simulink model "L1_CBF_ACC"  (R2018a)
settings: Solver=FixedStepAuto  StartTime=0.0  StopTime=Tsim  FixedStep=0.001  RelTol=1e-3
InitFcn:
  | tic;
  | disp('Simulation started...');
  | L1_CBF_ACC
StopFcn:
  | elapsedTime_L1 = toc; % Stop timer when simulation ends
  | fprintf('Simulation Time: %.6f seconds\n', elapsedTime_L1);
  | 
  | % out_L1 = out;
undefined symbols (not defined in the file): case_num, D0, epsilon, f0, f1, f2, g, gamma, GTP, k, k_fric, m, magnitude, omega0, p_omega, psc, v0, vd, x10, x20
libraries: Projection x2
settings Model: Creator=Administrator  LastModifiedBy=hieunguyen412
settings DataIOCC: ReturnWorkspaceOutputs=on
settings SFSimCC: SimUseLocalCustomCode=on
settings RTWCC: RTWUseLocalCustomCode=on

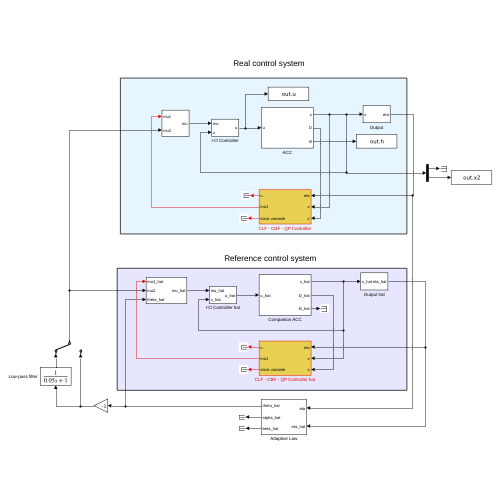
[thumbnail: Simulink's stored preview of the top-level diagram]
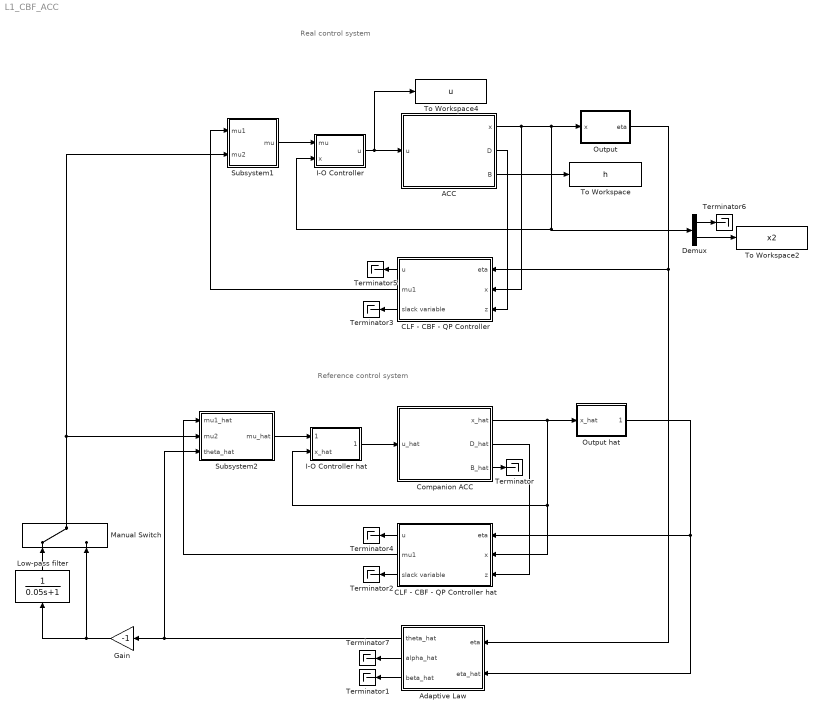
== system L1_CBF_ACC ==
  note: Real control system
  note: Reference control system
  ACC : Subsystem
  Adaptive Law : Subsystem
  CLF - CBF - QP Controller : Subsystem
  CLF - CBF - QP Controller hat : Subsystem
  Companion ACC : Subsystem
  Demux : Demux  Outputs=2
  Gain : Gain  Gain=-1
  I-O Controller : Subsystem
  I-O Controller hat : Subsystem
  Low-pass filter : TransferFcn  Denominator=[0.05 1]
  Manual Switch : ManualSwitch
  Output : Subsystem
  Output hat : Subsystem
  Subsystem1 : Subsystem
  Subsystem2 : Subsystem
  Terminator{,1..7} (8 alike) : Terminator
  To Workspace : ToWorkspace  VariableName=h  SampleTime=-1
  To Workspace2 : ToWorkspace  VariableName=x2  SampleTime=-1
  To Workspace4 : ToWorkspace  VariableName=u  SampleTime=-1
  wires:
  ACC/1(x) -> CLF - CBF - QP Controller/2(x), I-O Controller/2(x), Demux/1, Output/1(x)
  Output/1(eta) -> Adaptive Law/1(eta), CLF - CBF - QP Controller/1(eta)
  I-O Controller/1(u) -> To Workspace4/1, ACC/1(u)
  Adaptive Law/2(alpha_hat) -> Terminator7/1
  Adaptive Law/3(beta_hat) -> Terminator1/1
  ACC/3(B) -> To Workspace/1
  CLF - CBF - QP Controller/3(slack variable) -> Terminator3/1
  CLF - CBF - QP Controller/1(u) -> Terminator5/1
  ACC/2(D) -> CLF - CBF - QP Controller/3(z)
  Demux/2 -> To Workspace2/1
  Demux/1 -> Terminator6/1
  Subsystem1/1(mu) -> I-O Controller/1(mu)
  CLF - CBF - QP Controller/2(mu1) -> Subsystem1/1(mu1)
  CLF - CBF - QP Controller hat/2(mu1) -> Subsystem2/1(mu1_hat)
  Subsystem2/1(mu_hat) -> I-O Controller hat/1(mu_hat)
  Companion ACC/2(D_hat) -> CLF - CBF - QP Controller hat/3(z)
  CLF - CBF - QP Controller hat/1(u) -> Terminator4/1
  CLF - CBF - QP Controller hat/3(slack variable) -> Terminator2/1
  I-O Controller hat/1(u_hat) -> Companion ACC/1(u_hat)
  Output hat/1(eta_hat) -> Adaptive Law/2(eta_hat), CLF - CBF - QP Controller hat/1(eta)
  Companion ACC/1(x_hat) -> CLF - CBF - QP Controller hat/2(x), I-O Controller hat/2(x_hat), Output hat/1(x_hat)
  Low-pass filter/1 -> Manual Switch/1
  Gain/1 -> Low-pass filter/1, Manual Switch/2
  Manual Switch/1 -> Subsystem1/2(mu2), Subsystem2/2(mu2)
  Adaptive Law/1(theta_hat) -> Gain/1, Subsystem2/3(theta_hat)
  Companion ACC/3(B_hat) -> Terminator/1

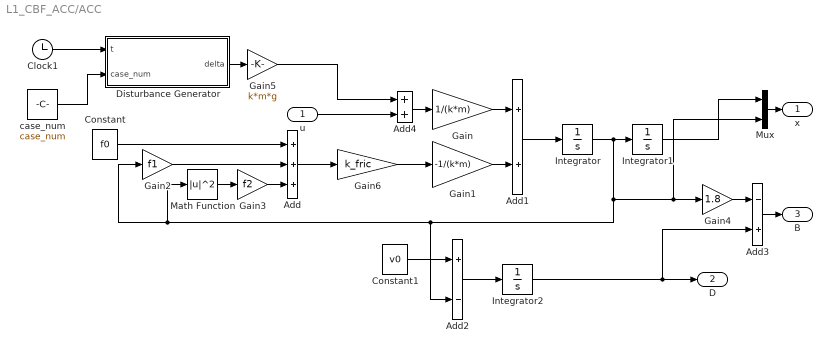
== system L1_CBF_ACC/ACC ==
  u : Inport  PortDimensions=1
  Add : Sum  Inputs=+++
  Add1 : Sum
  Add2 : Sum  Inputs=+-
  Add3 : Sum  Inputs=-+
  Add4 : Sum
  Clock1 : Clock
  Constant : Constant  Value=f0
  Constant1 : Constant  Value=v0
  Disturbance Generator : MATLAB Function  TreatAsAtomicUnit=on
  Gain : Gain  Gain=1/(k*m)
  Gain1 : Gain  Gain=-1/(k*m)
  Gain2 : Gain  Gain=f1
  Gain3 : Gain  Gain=f2
  Gain4 : Gain  Gain=1.8
  Gain5 : Gain  Gain=k*m*g
  Gain6 : Gain  Gain=k_fric
  Integrator : Integrator  InitialCondition=x20
  Integrator1 : Integrator  InitialCondition=x10
  Integrator2 : Integrator  InitialCondition=D0
  Math Function : Math  Operator=magnitude^2  SaturateOnIntegerOverflow=on
  Mux : Mux  Inputs=2
  case_num : Constant  Value=case_num
  x : Outport  PortDimensions=2
  D : Outport  Port=2  PortDimensions=1
  B : Outport  Port=3  PortDimensions=1
  wires:
  Constant/1 -> Add/1
  Gain2/1 -> Add/2
  Gain3/1 -> Add/3
  Gain/1 -> Add1/1
  Gain1/1 -> Add1/2
  Add1/1 -> Integrator/1
  Integrator/1 -> Add2/2, Math Function/1, Gain2/1, Mux/2, Gain4/1, Integrator1/1
  Math Function/1 -> Gain3/1
  Constant1/1 -> Add2/1
  Add2/1 -> Integrator2/1
  Integrator2/1 -> Add3/2, D/1
  Gain4/1 -> Add3/1
  Add3/1 -> B/1
  Mux/1 -> x/1
  Integrator1/1 -> Mux/1
  Gain5/1 -> Add4/1
  Add4/1 -> Gain/1
  Add/1 -> Gain6/1
  Gain6/1 -> Gain1/1
  u/1 -> Add4/2
  case_num/1 -> Disturbance Generator/2(case_num)
  Clock1/1 -> Disturbance Generator/1(t)
  Disturbance Generator/1(delta) -> Gain5/1

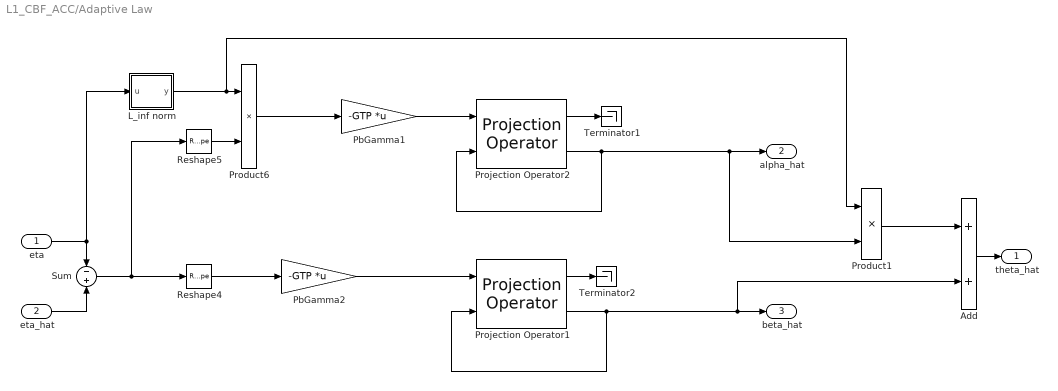
== system L1_CBF_ACC/Adaptive Law ==
  eta : Inport
  eta_hat : Inport  Port=2
  Add : Sum
  L_inf norm : MATLAB Function  TreatAsAtomicUnit=on
  PbGamma1 : Gain  Gain=-GTP  Multiplication=Matrix(K*u) (u vector)
  PbGamma2 : Gain  Gain=-GTP  Multiplication=Matrix(K*u) (u vector)
  Product1 : Product  RndMeth=Zero
  Product6 : Product  RndMeth=Zero
  Projection Operator1 : Projection/Projection Operator  EpsilonTheta=epsilon_beta  Prmax=beta_max  Prcenter=0  Pr0=0
  Projection Operator2 : Projection/Projection Operator  EpsilonTheta=epsilon_alpha  Prmax=alpha_max  Prcenter=0  Pr0=0
  Reshape4 : Reshape  OutputDimensionality=Row vector (2-D)
  Reshape5 : Reshape  OutputDimensionality=Row vector (2-D)
  Sum : Sum  Inputs=-+
  Terminator1 : Terminator
  Terminator2 : Terminator
  theta_hat : Outport
  alpha_hat : Outport  Port=2
  beta_hat : Outport  Port=3
  wires:
  Reshape4/1 -> PbGamma2/1
  Reshape5/1 -> Product6/2
  Projection Operator2/1 -> Terminator1/1
  Sum/1 -> Reshape5/1, Reshape4/1
  eta_hat/1 -> Sum/2
  Projection Operator1/1 -> Terminator2/1
  Projection Operator2/2 -> Product1/2, alpha_hat/1, Projection Operator2/2
  Projection Operator1/2 -> Projection Operator1/2, Add/2, beta_hat/1
  PbGamma2/1 -> Projection Operator1/1
  PbGamma1/1 -> Projection Operator2/1
  Product6/1 -> PbGamma1/1
  eta/1 -> Sum/1, L_inf norm/1(u)
  L_inf norm/1(y) -> Product1/1, Product6/1
  Product1/1 -> Add/1
  Add/1 -> theta_hat/1

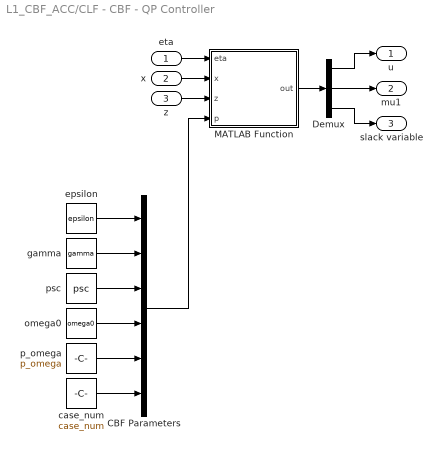
== system L1_CBF_ACC/CLF - CBF - QP Controller ==
  eta : Inport  PortDimensions=1
  x : Inport  Port=2  PortDimensions=2
  z : Inport  Port=3  PortDimensions=1
  CBF Parameters : Mux  Inputs=6
  Demux : Demux  Outputs=3
  MATLAB Function : MATLAB Function  TreatAsAtomicUnit=on  SystemSampleTime=0.001
  case_num : Constant  Value=case_num
  epsilon : Constant  Value=epsilon
  gamma : Constant  Value=gamma
  omega0 : Constant  Value=omega0
  p_omega : Constant  Value=p_omega
  psc : Constant  Value=psc
  u : Outport  PortDimensions=1
  mu1 : Outport  Port=2  PortDimensions=1
  slack variable : Outport  Port=3  PortDimensions=1
  wires:
  Demux/1 -> u/1
  MATLAB Function/1(out) -> Demux/1
  Demux/3 -> slack variable/1
  Demux/2 -> mu1/1
  eta/1 -> MATLAB Function/1(eta)
  x/1 -> MATLAB Function/2(x)
  z/1 -> MATLAB Function/3(z)
  gamma/1 -> CBF Parameters/2
  omega0/1 -> CBF Parameters/4
  epsilon/1 -> CBF Parameters/1
  p_omega/1 -> CBF Parameters/5
  psc/1 -> CBF Parameters/3
  CBF Parameters/1 -> MATLAB Function/4(p)
  case_num/1 -> CBF Parameters/6

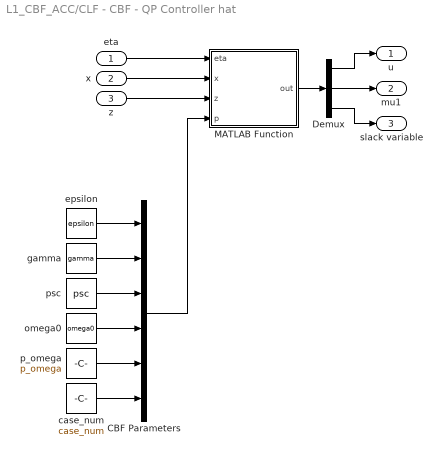
== system L1_CBF_ACC/CLF - CBF - QP Controller hat ==
  eta : Inport  PortDimensions=1
  x : Inport  Port=2  PortDimensions=2
  z : Inport  Port=3  PortDimensions=1
  CBF Parameters : Mux  Inputs=6
  Demux : Demux  Outputs=3
  MATLAB Function : MATLAB Function  TreatAsAtomicUnit=on  SystemSampleTime=0.001
  case_num : Constant  Value=case_num
  epsilon : Constant  Value=epsilon
  gamma : Constant  Value=gamma
  omega0 : Constant  Value=omega0
  p_omega : Constant  Value=p_omega
  psc : Constant  Value=psc
  u : Outport  PortDimensions=1
  mu1 : Outport  Port=2  PortDimensions=1
  slack variable : Outport  Port=3  PortDimensions=1
  wires:
  x/1 -> MATLAB Function/2(x)
  z/1 -> MATLAB Function/3(z)
  eta/1 -> MATLAB Function/1(eta)
  Demux/3 -> slack variable/1
  Demux/2 -> mu1/1
  MATLAB Function/1(out) -> Demux/1
  Demux/1 -> u/1
  case_num/1 -> CBF Parameters/6
  CBF Parameters/1 -> MATLAB Function/4(p)
  p_omega/1 -> CBF Parameters/5
  epsilon/1 -> CBF Parameters/1
  omega0/1 -> CBF Parameters/4
  psc/1 -> CBF Parameters/3
  gamma/1 -> CBF Parameters/2

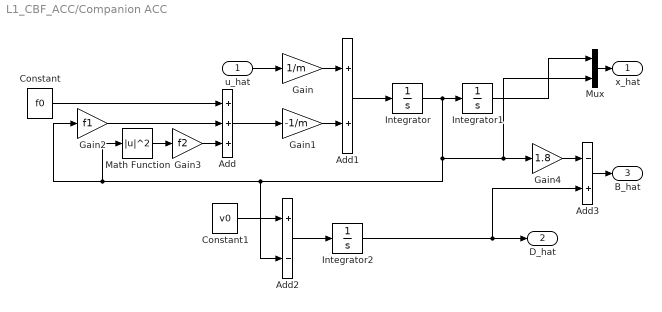
== system L1_CBF_ACC/Companion ACC ==
  u_hat : Inport  PortDimensions=1
  Add : Sum  Inputs=+++
  Add1 : Sum
  Add2 : Sum  Inputs=+-
  Add3 : Sum  Inputs=-+
  Constant : Constant  Value=f0
  Constant1 : Constant  Value=v0
  Gain : Gain  Gain=1/m
  Gain1 : Gain  Gain=-1/m
  Gain2 : Gain  Gain=f1
  Gain3 : Gain  Gain=f2
  Gain4 : Gain  Gain=1.8
  Integrator : Integrator  InitialCondition=x20
  Integrator1 : Integrator  InitialCondition=x10
  Integrator2 : Integrator  InitialCondition=D0
  Math Function : Math  Operator=magnitude^2  SaturateOnIntegerOverflow=on
  Mux : Mux  Inputs=2
  x_hat : Outport  PortDimensions=2
  D_hat : Outport  Port=2  PortDimensions=1
  B_hat : Outport  Port=3  PortDimensions=1
  wires:
  Integrator1/1 -> Mux/1
  Mux/1 -> x_hat/1
  Add3/1 -> B_hat/1
  Gain4/1 -> Add3/1
  Integrator2/1 -> D_hat/1, Add3/2
  Add2/1 -> Integrator2/1
  Constant1/1 -> Add2/1
  Math Function/1 -> Gain3/1
  Integrator/1 -> Mux/2, Gain4/1, Gain2/1, Math Function/1, Add2/2, Integrator1/1
  Add1/1 -> Integrator/1
  Gain1/1 -> Add1/2
  Gain/1 -> Add1/1
  u_hat/1 -> Gain/1
  Gain3/1 -> Add/3
  Gain2/1 -> Add/2
  Constant/1 -> Add/1
  Add/1 -> Gain1/1

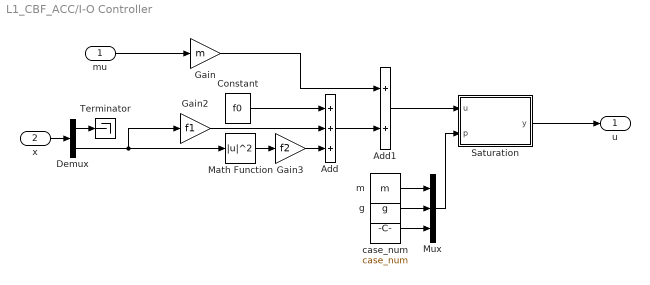
== system L1_CBF_ACC/I-O Controller ==
  mu : Inport
  x : Inport  Port=2  PortDimensions=2
  Add : Sum  Inputs=+++
  Add1 : Sum
  Constant : Constant  Value=f0
  Demux : Demux  Outputs=2
  Gain : Gain  Gain=m
  Gain2 : Gain  Gain=f1
  Gain3 : Gain  Gain=f2
  Math Function : Math  Operator=magnitude^2  SaturateOnIntegerOverflow=on
  Mux : Mux  Inputs=3
  Saturation : MATLAB Function  TreatAsAtomicUnit=on
  Terminator : Terminator
  case_num : Constant  Value=case_num
  g : Constant  Value=g
  m : Constant  Value=m
  u : Outport  PortDimensions=1
  wires:
  Gain3/1 -> Add/3
  Constant/1 -> Add/1
  Math Function/1 -> Gain3/1
  Gain2/1 -> Add/2
  Add/1 -> Add1/2
  mu/1 -> Gain/1
  Gain/1 -> Add1/1
  x/1 -> Demux/1
  Demux/2 -> Math Function/1, Gain2/1
  Demux/1 -> Terminator/1
  Add1/1 -> Saturation/1(u)
  Saturation/1(y) -> u/1
  case_num/1 -> Mux/3
  Mux/1 -> Saturation/2(p)
  g/1 -> Mux/2
  m/1 -> Mux/1

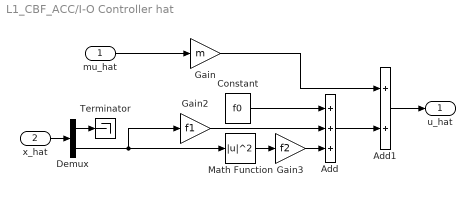
== system L1_CBF_ACC/I-O Controller hat ==
  mu_hat : Inport
  x_hat : Inport  Port=2  PortDimensions=2
  Add : Sum  Inputs=+++
  Add1 : Sum
  Constant : Constant  Value=f0
  Demux : Demux  Outputs=2
  Gain : Gain  Gain=m
  Gain2 : Gain  Gain=f1
  Gain3 : Gain  Gain=f2
  Math Function : Math  Operator=magnitude^2  SaturateOnIntegerOverflow=on
  Terminator : Terminator
  u_hat : Outport  PortDimensions=1
  wires:
  Demux/1 -> Terminator/1
  Demux/2 -> Gain2/1, Math Function/1
  x_hat/1 -> Demux/1
  Add1/1 -> u_hat/1
  Gain/1 -> Add1/1
  mu_hat/1 -> Gain/1
  Add/1 -> Add1/2
  Gain2/1 -> Add/2
  Math Function/1 -> Gain3/1
  Constant/1 -> Add/1
  Gain3/1 -> Add/3

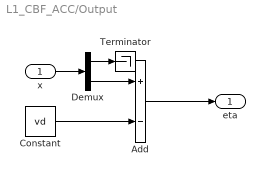
== system L1_CBF_ACC/Output ==
  x : Inport  PortDimensions=2
  Add : Sum  Inputs=+-
  Constant : Constant  Value=vd
  Demux : Demux  Outputs=2
  Terminator : Terminator
  eta : Outport  PortDimensions=1
  wires:
  Constant/1 -> Add/2
  Add/1 -> eta/1
  Demux/2 -> Add/1
  x/1 -> Demux/1
  Demux/1 -> Terminator/1

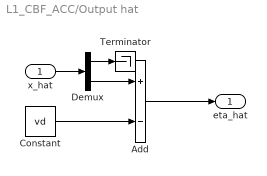
== system L1_CBF_ACC/Output hat ==
  x_hat : Inport  PortDimensions=2
  Add : Sum  Inputs=+-
  Constant : Constant  Value=vd
  Demux : Demux  Outputs=2
  Terminator : Terminator
  eta_hat : Outport  PortDimensions=1
  wires:
  Demux/1 -> Terminator/1
  x_hat/1 -> Demux/1
  Demux/2 -> Add/1
  Add/1 -> eta_hat/1
  Constant/1 -> Add/2

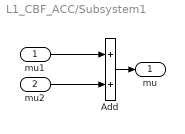
== system L1_CBF_ACC/Subsystem1 ==
  mu1 : Inport
  mu2 : Inport  Port=2
  Add : Sum
  mu : Outport
  wires:
  mu1/1 -> Add/1
  mu2/1 -> Add/2
  Add/1 -> mu/1

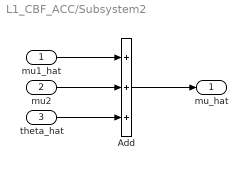
== system L1_CBF_ACC/Subsystem2 ==
  mu1_hat : Inport
  mu2 : Inport  Port=2
  theta_hat : Inport  Port=3
  Add : Sum  Inputs=+++
  mu_hat : Outport
  wires:
  theta_hat/1 -> Add/3
  mu2/1 -> Add/2
  mu1_hat/1 -> Add/1
  Add/1 -> mu_hat/1

== matlab function L1_CBF_ACC/Adaptive Law/L_inf norm ==
  data: u input; y output
function y = fcn(u)

y = max(abs(u));

== matlab function L1_CBF_ACC/I-O Controller/Saturation ==
  data: u input; y output; p input
function y = fcn(u, p)

m = p(1);
g = p(2);
case_num = p(3);

if case_num == 1 || case_num == 2
    y = u;
else
    if u >= 0.3*m*g
        y = 0.3*m*g;
    elseif u <= -0.3*m*g
        y = -0.3*m*g;
    else
        y = u;
    end
end

end

== matlab function L1_CBF_ACC/CLF - CBF - QP Controller hat/MATLAB Function ==
  data: eta input; out output; x input; z input; p input
function out = QP_Controller(eta, x, z, p)
coder.extrinsic('quadprog');

out = zeros(3,1);

x2 = x(2); 

case_num = p(6);
if case_num == 1 || case_num == 2
    mode = 1;
else 
    mode = 2;
end

%% Physical parameters
m = 1650;
g = 9.81; 
f0 = 0.1;
f1 = 5;
f2 = 0.25;
vd = 24;
v0 =  13.89;

ca = 0.3;
cd = 0.3;

%% Controller parameters
epsilon = p(1); 
gamma = p(2);
psc = p(3);
omega0 = p(4); 
p_omega = p(5);

%% Aerodynamic drag force
Fr = f0 + f1*x2 + f2*x2.^2;

%% ============== QP 1 (No input saturation) ==============
if mode == 1
    %% CLF
    y = eta;
    V = y^2;
    LfV = 2*y*(-Fr/m); LgV = 2*y/m;
    A_clf = [LgV 0 -1]; b_clf = -LfV -epsilon*V;
    
    %% CBF
    B = z - 1.8*x2;
    LfB = v0 - x2 + 1.8*Fr/m;
    LgB = -1.8/m;
    A_cbf = [-LgB, 0, 0]; b_cbf = LfB + gamma*B;
    
    %% I-O L
    Lfy = -Fr/m; Lgy = 1/m;
    A_iol = [Lgy -1 0]; b_iol = - Lfy;
    
    %% QP
    A_ieq = [A_clf; A_cbf]; b_ieq = [b_clf; b_cbf];
    
    A_eq = A_iol; b_eq = b_iol;
    
    H_acc = [0, 0, 0; 0, 1, 0; 0, 0, psc];
    F_acc = [0; 0; 0];
    
    U = quadprog(H_acc, F_acc, A_ieq, b_ieq, A_eq, b_eq);
    
    out = U([1 2 3]);
end
%% ============== QP 2 (Optimal-decay variable included for handling input saturation) ==============
if mode == 2
    %============= CLF ============
    y = eta;
    V = y^2;
    LfV = 2*y*(-Fr/m); LgV = 2*y/m;
    A_clf = [LgV 0 -1 0]; b_clf = -LfV -epsilon*V;
    
    %============= CBF 1 ============
    h1 = z - 1.8*x2;
    Lfh1 = v0 - x2 + 1.8*Fr/m; Lgh1 = -1.8/m;
    A_cbf1 = [-Lgh1 0 0 -gamma*h1]; b_cbf1 = Lfh1 + omega0*gamma*h1;
    
    %============= I-O L ============
    Lfy = -Fr/m; Lgy = 1/m;
    A_iol = [Lgy -1 0 0]; b_iol = - Lfy;
    
    %============= Input constraints ============
    umax = ca*m*g; umin = -cd*m*g;
    A_ic = [1 0 0 0; -1 0 0 0]; b_ic = [umax; -umin];
    
    %============= QP ============
    H_acc = [0, 0, 0, 0; 0, 1, 0, 0; 0, 0, psc, 0; 0, 0, 0, p_omega];
    F_acc = [0; 0; 0; 0];
    
    A_ieq = [A_clf; A_cbf1; A_ic]; b_ieq = [b_clf; b_cbf1; b_ic];
    
    A_eq = A_iol; b_eq = b_iol;
    
    U = quadprog(H_acc, F_acc, A_ieq, b_ieq, A_eq, b_eq);

    out = U([1 2 3]);
end

end

== matlab function L1_CBF_ACC/CLF - CBF - QP Controller/MATLAB Function ==
  data: eta input; out output; x input; z input; p input
function out = QP_Controller(eta, x, z, p)
coder.extrinsic('quadprog');

out = zeros(3,1);

x2 = x(2); 

case_num = p(6);
if case_num == 1 || case_num == 2
    mode = 1;
else 
    mode = 2;
end

%% Physical parameters
m = 1650;
g = 9.81; 
f0 = 0.1;
f1 = 5;
f2 = 0.25;
vd = 24;
v0 =  13.89;

ca = 0.3;
cd = 0.3;

%% Controller parameters
epsilon = p(1); 
gamma = p(2);
psc = p(3);
omega0 = p(4); 
p_omega = p(5);

%% Aerodynamic drag force
Fr = f0 + f1*x2 + f2*x2.^2;

%% ============== QP 1 (No input saturation) ==============
if mode == 1
    %% CLF
    y = eta;
    V = y^2;
    LfV = 2*y*(-Fr/m); LgV = 2*y/m;
    A_clf = [LgV 0 -1]; b_clf = -LfV -epsilon*V;
    
    %% CBF
    B = z - 1.8*x2;
    LfB = v0 - x2 + 1.8*Fr/m;
    LgB = -1.8/m;
    A_cbf = [-LgB, 0, 0]; b_cbf = LfB + gamma*B;
    
    %% I-O L
    Lfy = -Fr/m; Lgy = 1/m;
    A_iol = [Lgy -1 0]; b_iol = - Lfy;
    
    %% QP
    A_ieq = [A_clf; A_cbf]; b_ieq = [b_clf; b_cbf];
    
    A_eq = A_iol; b_eq = b_iol;
    
    H_acc = [0, 0, 0; 0, 1, 0; 0, 0, psc];
    F_acc = [0; 0; 0];
    
    U = quadprog(H_acc, F_acc, A_ieq, b_ieq, A_eq, b_eq);
    
    out = U([1 2 3]);
end
%% ============== QP 2 (Optimal-decay variable included for handling input saturation) ==============
if mode == 2
    %============= CLF ============
    y = eta;
    V = y^2;
    LfV = 2*y*(-Fr/m); LgV = 2*y/m;
    A_clf = [LgV 0 -1 0]; b_clf = -LfV -epsilon*V;
    
    %============= CBF 1 ============
    h1 = z - 1.8*x2;
    Lfh1 = v0 - x2 + 1.8*Fr/m; Lgh1 = -1.8/m;
    A_cbf1 = [-Lgh1 0 0 -gamma*h1]; b_cbf1 = Lfh1 + omega0*gamma*h1;
    
    %============= I-O L ============
    Lfy = -Fr/m; Lgy = 1/m;
    A_iol = [Lgy -1 0 0]; b_iol = - Lfy;
    
    %============= Input constraints ============
    umax = ca*m*g; umin = -cd*m*g;
    A_ic = [1 0 0 0; -1 0 0 0]; b_ic = [umax; -umin];
    
    %============= QP ============
    H_acc = [0, 0, 0, 0; 0, 1, 0, 0; 0, 0, psc, 0; 0, 0, 0, p_omega];
    F_acc = [0; 0; 0; 0];
    
    A_ieq = [A_clf; A_cbf1; A_ic]; b_ieq = [b_clf; b_cbf1; b_ic];
    
    A_eq = A_iol; b_eq = b_iol;
    
    U = quadprog(H_acc, F_acc, A_ieq, b_ieq, A_eq, b_eq);

    out = U([1 2 3]);
end


end

== matlab function L1_CBF_ACC/ACC/Disturbance Generator ==
  data: t input; delta output; case_num input
function delta = fcn(t, case_num)

if case_num == 1
    delta = 0.16*cos(2*pi*t/20) + 0.14*sin(2*pi*t/10 + pi/3);
elseif case_num == 2
    delta = 0.16*cos(2*pi*t/20) + 0.14*sin(2*pi*t/10 + pi/3);
else
    % delta = 0.18*cos(2*pi*t/20) + 0.14*sin(2*pi*t/10 - pi/8);
    delta = -(0.12*cos(2*pi*t/20) + 0.08*sin(2*pi*t/10 + pi/3));
end
